simulink model "heading_loop"  (Simulink 7.4)
settings: Solver=ode45  StartTime=0.0  StopTime=100  RelTol=1e-3
values from neighbouring files (symbols this model uses):
  a_phi1 = den(2)    [computeGains.m]    (also in compute_tf_model.m = -0.5*rho*Va_trim^2*S_wing*b*C_p_p*b/2/Va_trim)
  a_phi2 = num(3)    [computeGains.m]    (also in compute_tf_model.m = 0.5*rho*Va_trim^2*S_wing*b*C_p_delta_a)
  delta_a_max = 45*pi/180    (= 0.785398163397)    [computeGains.m]
  P = varargin{5}    [my_mav_dynamics.m]
settings Model: Creator=beard  LastModifiedBy=beard

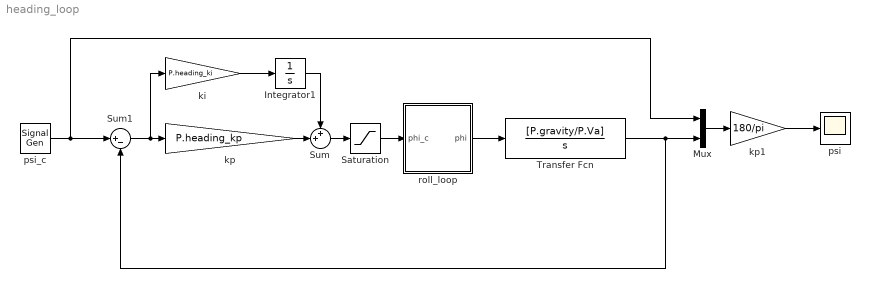
== system heading_loop ==
  Integrator1 : Integrator
  Mux : Mux  Inputs=2
  Saturation : Saturate  UpperLimit=30*pi/180  LowerLimit=-30*pi/180  OutDataType=fixdt(1, 16)  OutScaling=2^0
  Sum : Sum  Inputs=++|  OutDataType=fixdt(1, 16)  OutScaling=2^0
  Sum1 : Sum  Inputs=|+-  OutDataType=fixdt(1, 16)  OutScaling=2^0
  Transfer Fcn : TransferFcn  Numerator=[P.gravity/P.Va]  Denominator=[1 0]
  ki : Gain  Gain=P.heading_ki  ParameterDataType=fixdt(1, 16)  ParameterScaling=2^0  OutDataType=fixdt(1, 16)  OutScaling=2^0
  kp : Gain  Gain=P.heading_kp  ParameterDataType=fixdt(1, 16)  ParameterScaling=2^0  OutDataType=fixdt(1, 16)  OutScaling=2^0
  kp1 : Gain  Gain=180/pi  ParameterDataType=fixdt(1, 16)  ParameterScaling=2^0  OutDataType=fixdt(1, 16)  OutScaling=2^0
  psi : Scope
      settings: TimeRange=100  YMin=-40  YMax=60
  psi_c : SignalGenerator  WaveForm=square  Amplitude=25*pi/180  Frequency=.01
  roll_loop : Subsystem
  wires:
  Sum/1 -> Saturation/1
  kp/1 -> Sum/2
  Sum1/1 -> kp/1, ki/1
  ki/1 -> Integrator1/1
  Integrator1/1 -> Sum/1
  psi_c/1 -> Sum1/1, Mux/1
  kp1/1 -> psi/1
  Mux/1 -> kp1/1
  roll_loop/1(phi) -> Transfer Fcn/1
  Transfer Fcn/1 -> Mux/2, Sum1/2
  Saturation/1 -> roll_loop/1(phi_c)

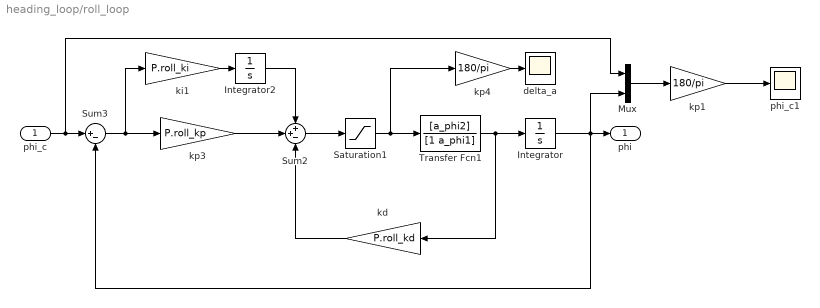
== system heading_loop/roll_loop ==
  phi_c : Inport
  Integrator : Integrator
  Integrator2 : Integrator
  Mux : Mux  Inputs=2
  Saturation1 : Saturate  UpperLimit=delta_a_max  LowerLimit=-delta_a_max  OutDataType=fixdt(1, 16)  OutScaling=2^0
  Sum2 : Sum  Inputs=++-  OutDataType=fixdt(1, 16)  OutScaling=2^0
  Sum3 : Sum  Inputs=|+-  OutDataType=fixdt(1, 16)  OutScaling=2^0
  Transfer Fcn1 : TransferFcn  Numerator=[a_phi2]  Denominator=[1 a_phi1]
  delta_a : Scope
      settings: TimeRange=100  YMin=-50  YMax=50  SaveName=ScopeData2
  kd : Gain  Gain=P.roll_kd  ParameterDataType=fixdt(1, 16)  ParameterScaling=2^0  OutDataType=fixdt(1, 16)  OutScaling=2^0
  ki1 : Gain  Gain=P.roll_ki  ParameterDataType=fixdt(1, 16)  ParameterScaling=2^0  OutDataType=fixdt(1, 16)  OutScaling=2^0
  kp1 : Gain  Gain=180/pi  ParameterDataType=fixdt(1, 16)  ParameterScaling=2^0  OutDataType=fixdt(1, 16)  OutScaling=2^0
  kp3 : Gain  Gain=P.roll_kp  ParameterDataType=fixdt(1, 16)  ParameterScaling=2^0  OutDataType=fixdt(1, 16)  OutScaling=2^0
  kp4 : Gain  Gain=180/pi  ParameterDataType=fixdt(1, 16)  ParameterScaling=2^0  OutDataType=fixdt(1, 16)  OutScaling=2^0
  phi_c1 : Scope
      settings: TimeRange=100  YMin=-30  YMax=40  SaveName=ScopeData3
  phi : Outport
  wires:
  Transfer Fcn1/1 -> Integrator/1, kd/1
  Saturation1/1 -> Transfer Fcn1/1, kp4/1
  Sum2/1 -> Saturation1/1
  kd/1 -> Sum2/3
  kp3/1 -> Sum2/2
  Sum3/1 -> kp3/1, ki1/1
  ki1/1 -> Integrator2/1
  Integrator2/1 -> Sum2/1
  Integrator/1 -> Sum3/2, phi/1, Mux/2
  kp4/1 -> delta_a/1
  phi_c/1 -> Sum3/1, Mux/1
  Mux/1 -> kp1/1
  kp1/1 -> phi_c1/1
